simulink model "Observers"  (R2020b)
settings: Solver=ode45  StartTime=0.0  StopTime=T  MaxStep=0.001  RelTol=1e-3
values from neighbouring files (symbols this model uses):
  alpha = mu_2*C    (= 62.8318530718)    [DifferentiatorParameter.m]    (also in Observer_parameter.m = [alpha_1, 2*alpha_1-1, alpha_2, 2*alpha_2-1]')
  Base_Obs = [1,0,0,0;0,0,1,0;0,1,0,0;0,0,0,1]    [Observer_parameter.m]
  C_obs = [C1_obs, zeros(1,2); zeros(1,2), C2_obs]    [Observer_parameter.m]
  K = place(A', C', [-5,-2])'./d    [DifferentiatorParameter.m]    (also in Observer_parameter.m = lqr(A, B, eye(4), 10); Project.m = lqr(A, B, eye(4), 2))
  K_HGO = [K1_HGO, zeros(2,1); zeros(2,1), K2_HGO]    [Observer_parameter.m]
  K_SM = [K1_SM, zeros(2,1); zeros(2,1), K2_SM]    [Observer_parameter.m]
  pendulumParameter_model_1 = PendulumParameter()    [Observer_parameter.m]
  T = 10    [DifferentiatorParameter.m]    (also in Observer_parameter.m; Project.m)
  Te = 1e-3    (= 0.001)    [DifferentiatorParameter.m]    (also in Observer_parameter.m; Project.m)
  X_eq = [0;pi;0;0]    [Observer_parameter.m]    (also in Project.m = [0;-pi;0;0])
undefined symbols (not defined in the file or in its folder): sigbuilder_block
libraries: simulink x1, powerlib_meascontrol x1, simulink_extras x1
settings Model: Creator=vorps  LastModifiedBy=vorps
settings SolverCC: ZeroCrossAlgorithm=Adaptive  AlgebraicLoopSolver=LineSearch
settings DebuggingCC: IgnoredZcDiagnostic=none

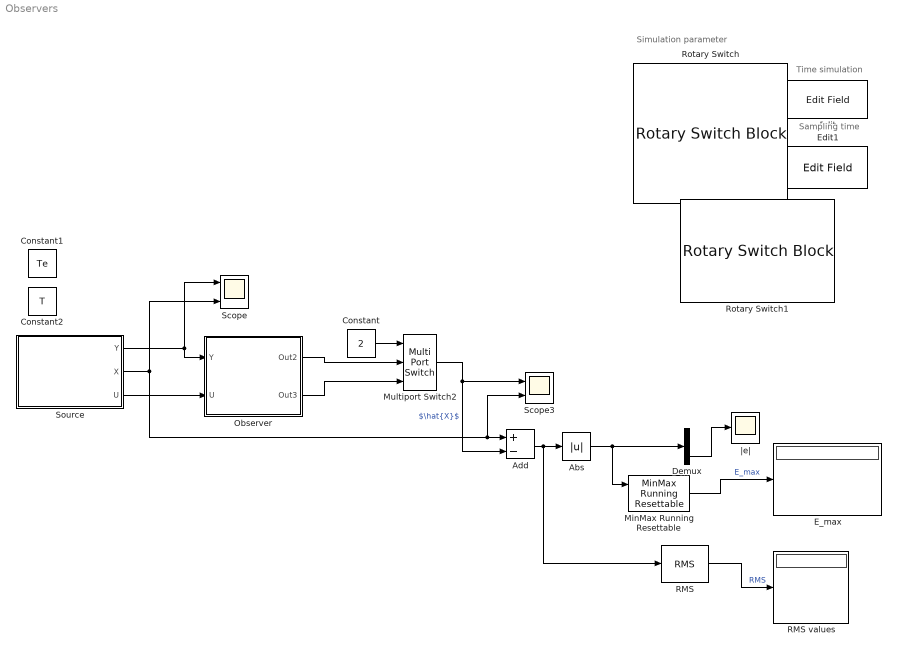
== system Observers ==
  note: Sampling time
  note: Time simulation
  note: Simulation parameter
  Abs : Abs  ZeroCross=off
  Add : Sum  Inputs=+-
  Constant : Constant  Value=2
  Constant1 : Constant  Value=Te
  Constant2 : Constant  Value=T
  Demux : Demux  Outputs=2
  E_max : Display
  Edit : EditField  ShowInitialText=on  Alignment=Left
  Edit1 : EditField  ShowInitialText=on  Alignment=Left
  MinMax Running Resettable : simulink/Math Operations/MinMax Running Resettable  Function=max  vinit=0.0
  Multiport Switch2 : MultiPortSwitch  Inputs=2  InputSameDT=on
  Observer : Subsystem
  RMS : powerlib_meascontrol/Measurements/RMS  TrueRMS=on  Freq=1/T  RMSInit=120  Ts=Te
  RMS values : Display
  Rotary Switch : RotarySwitchBlock
      settings: Values={{'HGO', 'Sliding mode'}, [1 2]}
  Rotary Switch1 : RotarySwitchBlock
      settings: Values={{'True model', 'Model 1'}, [1 2]}
  Scope : Scope  NumInputPorts=2
  Scope3 : Scope  NumInputPorts=2
  Source : Subsystem
  |e| : Scope
  wires:
  Source/2(X) -> Scope/2, Scope3/2, Add/1
  Source/1(Y) -> Scope/1, Observer/1(Y)
  Constant/1 -> Multiport Switch2/1
  Multiport Switch2/1 -> Add/2, Scope3/1  "$\\hat{X}$"
  Add/1 -> RMS/1, Abs/1
  Abs/1 -> MinMax Running Resettable/1, Demux/1
  RMS/1 -> RMS values/1  "RMS"
  MinMax Running Resettable/1 -> E_max/1  "E_max"
  Source/3(U) -> Observer/2(U)
  Observer/1(Out2) -> Multiport Switch2/2
  Observer/2(Out3) -> Multiport Switch2/3
  Demux/2 -> |e|/1

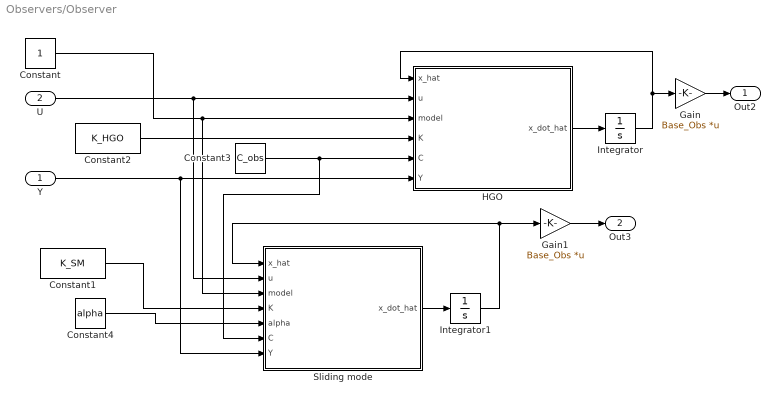
== system Observers/Observer ==
  Y : Inport
  U : Inport  Port=2
  Constant : Constant
  Constant1 : Constant  Value=K_SM
  Constant2 : Constant  Value=K_HGO
  Constant3 : Constant  Value=C_obs
  Constant4 : Constant  Value=alpha
  Gain : Gain  Gain=Base_Obs  Multiplication=Matrix(K*u)
  Gain1 : Gain  Gain=Base_Obs  Multiplication=Matrix(K*u)
  HGO : MATLAB Function  TreatAsAtomicUnit=on
  Integrator : Integrator  InitialCondition=zeros(4,1)
  Integrator1 : Integrator  InitialCondition=zeros(4,1)
  Sliding mode : MATLAB Function  TreatAsAtomicUnit=on
  Out2 : Outport
  Out3 : Outport  Port=2
  wires:
  Y/1 -> Sliding mode/7(Y), HGO/6(Y)
  Sliding mode/1(x_dot_hat) -> Integrator1/1
  Constant2/1 -> HGO/4(K)
  Constant3/1 -> Sliding mode/6(C), HGO/5(C)
  Constant4/1 -> Sliding mode/5(alpha)
  Integrator1/1 -> Gain1/1, Sliding mode/1(x_hat)
  HGO/1(x_dot_hat) -> Integrator/1
  Integrator/1 -> HGO/1(x_hat), Gain/1
  Gain1/1 -> Out3/1
  U/1 -> Sliding mode/2(u), HGO/2(u)
  Constant/1 -> Sliding mode/3(model), HGO/3(model)
  Gain/1 -> Out2/1
  Constant1/1 -> Sliding mode/4(K)

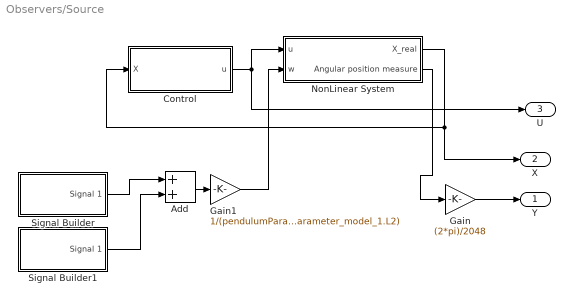
== system Observers/Source ==
  Add : Sum
  Control : Subsystem
  Gain : Gain  Gain=(2*pi)/2048
  Gain1 : Gain  Gain=1/(pendulumParameter_model_1.M2*pendulumParameter_model_1.L2)
  NonLinear System : Subsystem
  Signal Builder : Subsystem  Tag=STV Subsys  LoadFcn=sigbuilder_block('load');  StartFcn=sigbuilder_block('start');  StopFcn=sigbuilder_block('stop');  ClipboardFcn=sigbuilder_block('clipboard');  mask(Sigbuilder block){tuvar=[0:10]}
      mask help: Simulink:masks:SigbuilderBlock_MD
      mask init:
      | if ~strcmp(get_param(bdroot(gcbh),'SimulationStatus'),'stopped') tuvar = sigbuilder_block('maskInit'); end
      settings: CopyFcn=sigbuilder_block('copy');  DeleteFcn=sigbuilder_block('delete');  ModelCloseFcn=sigbuilder_block('modelClose');  PreSaveFcn=sigbuilder_block('preSave');  PauseFcn=sigbuilder_block('pause');  ContinueFcn=sigbuilder_block('continue');  NameChangeFcn=sigbuilder_block('namechange');  OpenFcn=sigbuilder_block('open',[886.5 189.75 550.5 358.5 ]);  CloseFcn=sigbuilder_block('close');
      mask Display: plot(0, 0, 100, 100,[2, 2, 32, 32, 2], [68, 8, 8, 68, 68],[32, 2], [38, 38], [32, 19, 2],[53, 60, 44], [32, 17, 17, 2],[16, 16, 31, 31]);txt = getActiveGroup(gcbh);text(2, 100, txt,'verticalAlignment', 'top');
  Signal Builder1 : Subsystem  Tag=STV Subsys  LoadFcn=sigbuilder_block('load');  StartFcn=sigbuilder_block('start');  StopFcn=sigbuilder_block('stop');  ClipboardFcn=sigbuilder_block('clipboard');  mask(Sigbuilder block){tuvar=[0:10]}
      mask help: Simulink:masks:SigbuilderBlock_MD
      mask init:
      | if ~strcmp(get_param(bdroot(gcbh),'SimulationStatus'),'stopped') tuvar = sigbuilder_block('maskInit'); end
      settings: CopyFcn=sigbuilder_block('copy');  DeleteFcn=sigbuilder_block('delete');  ModelCloseFcn=sigbuilder_block('modelClose');  PreSaveFcn=sigbuilder_block('preSave');  PauseFcn=sigbuilder_block('pause');  ContinueFcn=sigbuilder_block('continue');  NameChangeFcn=sigbuilder_block('namechange');  OpenFcn=sigbuilder_block('open',[843.75 185.25 550.5 358.5 ]);  CloseFcn=sigbuilder_block('close');
      mask Display: plot(0, 0, 100, 100,[2, 2, 32, 32, 2], [68, 8, 8, 68, 68],[32, 2], [38, 38], [32, 19, 2],[53, 60, 44], [32, 17, 17, 2],[16, 16, 31, 31]);txt = getActiveGroup(gcbh);text(2, 100, txt,'verticalAlignment', 'top');
  Y : Outport
  X : Outport  Port=2
  U : Outport  Port=3
  wires:
  NonLinear System/1(X_real) -> X/1, Control/1(X)
  NonLinear System/2(Angular position measure) -> Gain/1
  Gain/1 -> Y/1
  Control/1(u) -> U/1, NonLinear System/1(u)
  Signal Builder1/1(Signal 1) -> Add/2
  Add/1 -> Gain1/1
  Signal Builder/1(Signal 1) -> Add/1
  Gain1/1 -> NonLinear System/2(w)

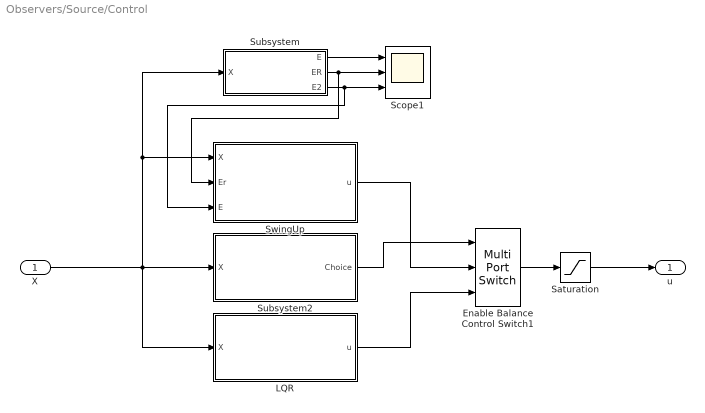
== system Observers/Source/Control ==
  X : Inport
  Enable Balance Control Switch1 : MultiPortSwitch  DataPortOrder=Zero-based contiguous  Inputs=2  zeroidx=on
  LQR : Subsystem
  Saturation : Saturate  UpperLimit=10  LowerLimit=-10
  Scope1 : Scope  NumInputPorts=3
  Subsystem : Subsystem
  Subsystem2 : Subsystem
  SwingUp : Subsystem
  u : Outport
  wires:
  LQR/1(u) -> Enable Balance Control Switch1/3
  Subsystem/2(ER) -> SwingUp/2(Er), Scope1/2
  Subsystem/1(E) -> Scope1/1
  SwingUp/1(u) -> Enable Balance Control Switch1/2
  Subsystem/3(E2) -> SwingUp/3(E), Scope1/3
  X/1 -> Subsystem/1(X), SwingUp/1(X), Subsystem2/1(X), LQR/1(X)
  Subsystem2/1(Choice) -> Enable Balance Control Switch1/1
  Enable Balance Control Switch1/1 -> Saturation/1
  Saturation/1 -> u/1

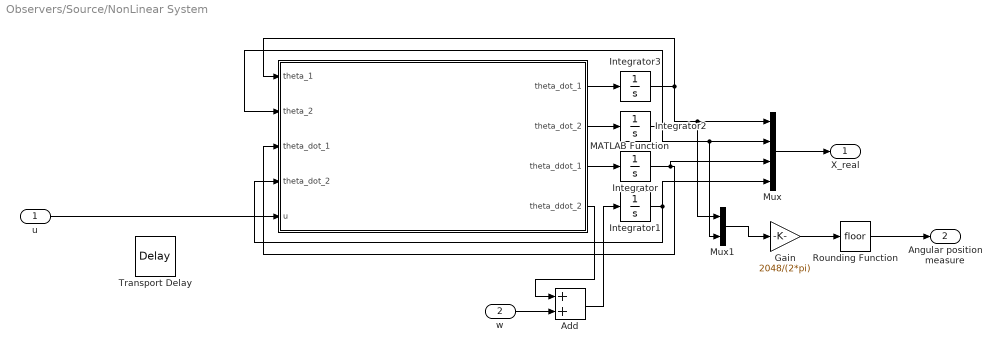
== system Observers/Source/NonLinear System ==
  u : Inport
  w : Inport  Port=2
  Add : Sum
  Gain : Gain  Gain=2048/(2*pi)
  Integrator : Integrator
  Integrator1 : Integrator
  Integrator2 : Integrator  InitialCondition=0.1
  Integrator3 : Integrator
  MATLAB Function : MATLAB Function  TreatAsAtomicUnit=on
  Mux : Mux
  Mux1 : Mux  Inputs=2
  Rounding Function : Rounding
  Transport Delay : TransportDelay  DelayTime=0.02
  X_real : Outport
  Angular position measure : Outport  Port=2
  wires:
  Mux/1 -> X_real/1
  Integrator3/1 -> MATLAB Function/1(theta_1), Mux/1, Mux1/1
  Integrator1/1 -> MATLAB Function/4("theta_dot_2 "), Mux/4
  Integrator2/1 -> MATLAB Function/2(theta_2), Mux1/2, Mux/2
  Integrator/1 -> Mux/3, MATLAB Function/3("theta_dot_1 ")
  MATLAB Function/3(theta_ddot_1) -> Integrator/1
  MATLAB Function/1(theta_dot_1) -> Integrator3/1
  Gain/1 -> Rounding Function/1
  Rounding Function/1 -> Angular position measure/1
  Mux1/1 -> Gain/1
  w/1 -> Add/2
  MATLAB Function/2(theta_dot_2) -> Integrator2/1
  MATLAB Function/4(theta_ddot_2) -> Add/1
  Add/1 -> Integrator1/1
  u/1 -> MATLAB Function/5(u)

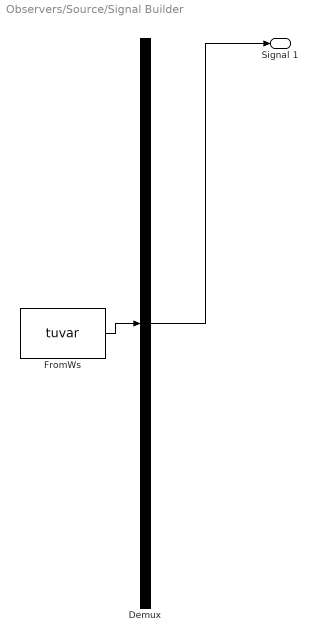
== system Observers/Source/Signal Builder ==
  Demux : Demux  Tag=STV Demux  Outputs=1
      settings: DisplayOption=none
  FromWs : FromWorkspace  Tag=STV FromWs  VariableName=tuvar
      SigBuilderData=|
      | common.afterFinalStr = 'Extrapolate'
      | common.sampleTime = 0
      | dataSet.timeRange = [0 10]
      | dataSet.name = 'Group 1'
      | sbobj.Groups.Name = 'Group 1'
      | sbobj.Groups.Signals.Name = 'Signal 1'
      | sbobj.Groups.Signals.XData = [0 4 4.2 4.2 10]
      | sbobj.Groups.Signals.YData = [0 0 0.2 0 0]
  Signal 1 : Outport  Tag=STV Outport
  wires:
  Demux/1 -> Signal 1/1
  FromWs/1 -> Demux/1

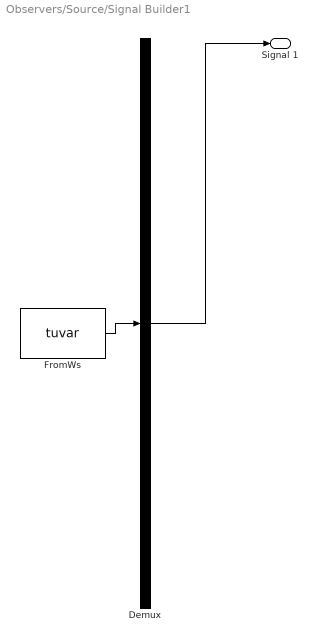
== system Observers/Source/Signal Builder1 ==
  Demux : Demux  Tag=STV Demux  Outputs=1
      settings: DisplayOption=none
  FromWs : FromWorkspace  Tag=STV FromWs  VariableName=tuvar
      SigBuilderData=|
      | common.afterFinalStr = 'Extrapolate'
      | common.sampleTime = 0
      | dataSet.timeRange = [0 10]
      | dataSet.name = 'Group 1'
      | sbobj.Groups.Name = 'Group 1'
      | sbobj.Groups.Signals.Name = 'Signal 1'
      | sbobj.Groups.Signals.XData = [0 6.5 6.7 6.7 10]
      | sbobj.Groups.Signals.YData = [0 0 0.3 0 0]
  Signal 1 : Outport  Tag=STV Outport
  wires:
  Demux/1 -> Signal 1/1
  FromWs/1 -> Demux/1

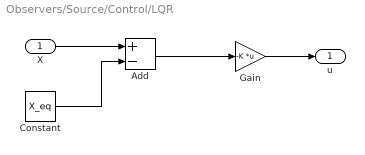
== system Observers/Source/Control/LQR ==
  X : Inport
  Add : Sum  Inputs=+-
  Constant : Constant  Value=X_eq
  Gain : Gain  Gain=-K  Multiplication=Matrix(K*u)
  u : Outport
  wires:
  Add/1 -> Gain/1
  Constant/1 -> Add/2
  Gain/1 -> u/1
  X/1 -> Add/1

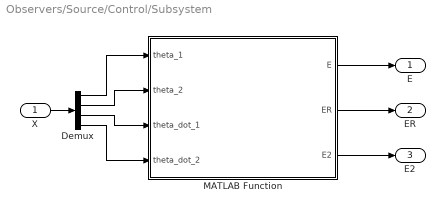
== system Observers/Source/Control/Subsystem ==
  X : Inport
  Demux : Demux
  MATLAB Function : MATLAB Function  TreatAsAtomicUnit=on
  E : Outport
  ER : Outport  Port=2
  E2 : Outport  Port=3
  wires:
  X/1 -> Demux/1
  Demux/1 -> MATLAB Function/1(theta_1)
  Demux/2 -> MATLAB Function/2(theta_2)
  Demux/3 -> MATLAB Function/3(theta_dot_1)
  Demux/4 -> MATLAB Function/4(theta_dot_2)
  MATLAB Function/1(E) -> E/1
  MATLAB Function/2(ER) -> ER/1
  MATLAB Function/3(E2) -> E2/1

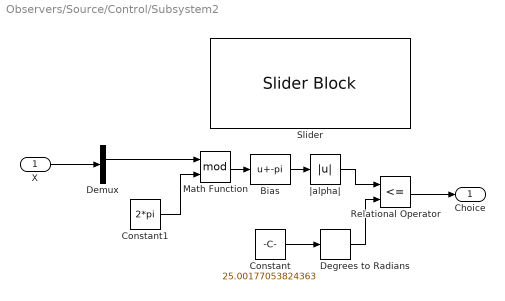
== system Observers/Source/Control/Subsystem2 ==
  X : Inport
  Bias : Bias  Bias=-pi
  Constant : Constant  Value=25.00177053824363
  Constant1 : Constant  Value=2*pi
  Degrees to Radians : simulink_extras/Transformations/Degrees to Radians
  Demux : Demux
  Math Function : Math  Operator=mod  SignedPower=on  SaturateOnIntegerOverflow=on
  Relational Operator : RelationalOperator  Operator=<=  OutDataTypeStr=boolean  RndMeth=Simplest
  Slider : SliderBlock  ScaleMax=180
  |alpha| : Abs
  Choice : Outport
  wires:
  X/1 -> Demux/1
  Math Function/1 -> Bias/1
  Demux/2 -> Math Function/1
  Relational Operator/1 -> Choice/1
  Constant1/1 -> Math Function/2
  Bias/1 -> |alpha|/1
  |alpha|/1 -> Relational Operator/1
  Constant/1 -> Degrees to Radians/1
  Degrees to Radians/1 -> Relational Operator/2

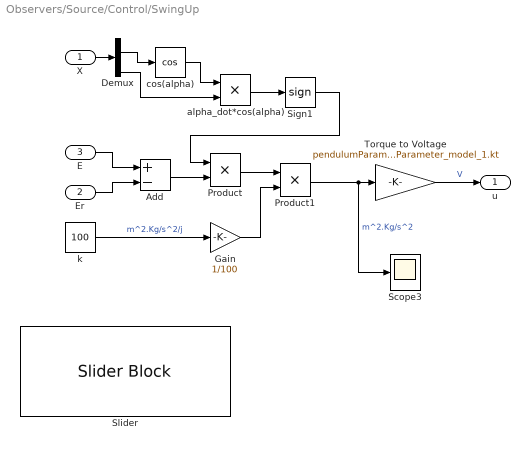
== system Observers/Source/Control/SwingUp ==
  X : Inport
  Er : Inport  Port=2
  E : Inport  Port=3
  Add : Sum  Inputs=+-
  Demux : Demux
  Gain : Gain  Gain=1/100
  Product : Product
  Product1 : Product
  Scope3 : Scope
  Sign1 : Signum  ZeroCross=off
  Slider : SliderBlock
  Torque to Voltage : Gain  Gain=pendulumParameter_model_1.Rm/pendulumParameter_model_1.kt
  alpha_dot*cos(alpha) : Product  RndMeth=Zero
  cos(alpha) : Trigonometry  Operator=cos
  k : Constant  Value=100
  u : Outport  VectorParamsAs1DForOutWhenUnconnected=off
  wires:
  X/1 -> Demux/1
  E/1 -> Add/1
  Er/1 -> Add/2
  cos(alpha)/1 -> alpha_dot*cos(alpha)/1
  Demux/2 -> cos(alpha)/1
  alpha_dot*cos(alpha)/1 -> Sign1/1
  Product/1 -> Product1/1
  k/1 -> Gain/1  "m^2.Kg/s^2/j"
  Demux/4 -> alpha_dot*cos(alpha)/2
  Product1/1 -> Scope3/1, Torque to Voltage/1  "m^2.Kg/s^2"
  Torque to Voltage/1 -> u/1  "V"
  Sign1/1 -> Product/1
  Add/1 -> Product/2
  Gain/1 -> Product1/2

== matlab function Observers/Source/Control/Subsystem/MATLAB Function ==
  data: theta_1 input; E output; theta_2 input; theta_dot_1 input; theta_dot_2 input; ER output; E2 output
function [E, ER, E2]  = energie(theta_1, theta_2, theta_dot_1, theta_dot_2)
    coder.extrinsic('evalin');
    pp = PendulumParameter();
    pp = evalin('base','pendulumParameter_model_1'); 
    E_p1 = 0;
    E_p2 = pp.g*pp.M2*pp.L2*(1-cos(theta_2))/2;
    E_k1 = 1/2*pp.J1*theta_dot_1^2;
    E_k2 = 1/2*theta_dot_1^2*(pp.M2*pp.L2^2+pp.J2*sin(theta_2)^2)+1/2*theta_dot_2^2*pp.J2 +pp.M2*pp.L1*pp.L2/2*cos(theta_2)*theta_dot_1*theta_dot_2;
    E = E_p1+E_p2+E_k1+E_k2;
    ER =pp.g*pp.M2*pp.L2;
    E2 = E_p2+theta_dot_2^2*pp.J2/2;
end

== matlab function Observers/Observer/HGO ==
  data: x_hat input; u input; model input; K input; x_dot_hat output; C input; Y input
function x_dot_hat = fcn(x_hat, u, model, K, C, Y)
    coder.extrinsic('evalin');
    coder.extrinsic('strcat');
    coder.extrinsic('num2str');
    number = num2str(model);
    pp = PendulumParameter();
    pp = evalin('base',strcat("pendulumParameter_model_", number));
    [f1,f2,f3,f4]=PendulumNonLinearModel(pp, x_hat(1),x_hat(3),x_hat(2),x_hat(4),u);
    x_dot_hat = [f1;f3;f2;f4]+K*(Y-C*x_hat);
end

== matlab function Observers/Source/NonLinear System/MATLAB Function ==
  data: theta_1 input; theta_2 input; theta_dot_1 input; theta_dot_2 input; u input; theta_dot_1 output; theta_dot_2 output; theta_ddot_1 output; theta_ddot_2 output
function [theta_dot_1,theta_dot_2,theta_ddot_1,theta_ddot_2]=PendulumNonLinearModel_internal(theta_1,theta_2,theta_dot_1,theta_dot_2,u)
    coder.extrinsic('evalin');
    pp = PendulumParameter();
    pp = evalin('base','pendulumParameter_model_1');
    [theta_dot_1,theta_dot_2,theta_ddot_1,theta_ddot_2]=PendulumNonLinearModel(pp, theta_1,theta_2,theta_dot_1,theta_dot_2,u);
end

== matlab function Observers/Observer/Sliding mode ==
  data: x_hat input; u input; model input; K input; x_dot_hat output; alpha input; C input; Y input
function x_dot_hat = fcn(x_hat, u, model, K, alpha, C, Y)
    coder.extrinsic('evalin');
    coder.extrinsic('strcat');
    coder.extrinsic('num2str');
    number = num2str(model);
    pp = PendulumParameter();
    pp = evalin('base',strcat("pendulumParameter_model_", number));
    [f1,f2,f3,f4]=PendulumNonLinearModel(pp, x_hat(1),x_hat(3),x_hat(2),x_hat(4),u);
    e = Y-C*x_hat;
    e_rep = repelem(e,2);
    x_dot_hat = [f1;f3;f2;f4]+K*sign(e).*(abs(e_rep).^alpha);
end
